simulink model "nonlinearrobot"  (R2020a)
settings: Solver=FixedStepDiscrete  StartTime=0.0  StopTime=1.5  FixedStep=1e-3  RelTol=1e-6  EnableMultiTasking=on
libraries: simulink x1
settings Model: Creator=amal029_old  LastModifiedBy=amal029_old
settings SolverCC: ZeroCrossAlgorithm=Adaptive  AutoInsertRateTranBlk=on  InsertRTBMode=Always
settings DataIOCC: LimitDataPoints=on  ReturnWorkspaceOutputs=off
settings OptimizationCC: LifeSpan=inf
settings DebuggingCC: AllowSymbolicDim=off  SFUnexpectedBacktrackingDiag=warning  SFNoUnconditionalDefaultTransitionDiag=warning  SFExecutionAtInitializationDiag=none  ArithmeticOperatorsInVariantConditions=warning
settings SFSimCC: SimUseLocalCustomCode=off  CustomCodeUndefinedFunction=UseInterfaceOnly
settings RTWCC: RTWUseLocalCustomCode=off
settings CodeAppCC: StateflowObjectComments=on
settings GRTTargetCC: TargetLangStandard=C89/C90 (ANSI)
settings ConfigComp: CovMetricSettings=dw  CovHtmlReporting=on  CovSaveCumulativeToWorkspaceVar=on  CovSaveSingleToWorkspaceVar=on  CovExternalEMLEnable=off  CovSFcnEnable=off

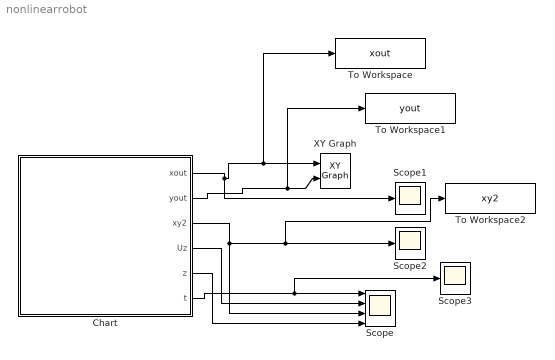
== system nonlinearrobot ==
  Chart : Stateflow chart  TreatAsAtomicUnit=on
  Scope : Scope  NumInputPorts=4
  Scope1 : Scope
  Scope2 : Scope
  Scope3 : Scope
  To Workspace : ToWorkspace  VariableName=xout  SampleTime=-1
  To Workspace1 : ToWorkspace  VariableName=yout  SampleTime=-1
  To Workspace2 : ToWorkspace  VariableName=xy2  SaveFormat=Structure With Time  SampleTime=-1
  XY Graph : simulink/Sinks/XY Graph  xmin=-5  xmax=5  ymin=-5  ymax=5  st=-1
  wires:
  Chart/1(xout) -> Scope1/1, To Workspace/1, XY Graph/1
  Chart/2(yout) -> To Workspace1/1, XY Graph/2
  Chart/3(xy2) -> To Workspace2/1, Scope2/1, Scope/3
  Chart/4(Uz) -> Scope/2
  Chart/5(z) -> Scope/4
  Chart/6(t) -> Scope3/1, Scope/1

== stateflow chart nonlinearrobot/Chart ==
  settings: sampleTime=1e-3
  state Changetheta
    du:
    t = t + v*D;
    z = z + (t)*D;
    en: -log(rand);
  note: This has different Wiener processes, because normrnd is being done separately.
      | These wiener processes are independent.
  state Inner
    du:
    x = x +v*cos(t)*D + v*normrnd(0, sqrt(D));
    y = y + v*sin(t)*D + v*normrnd(0, sqrt(D));
    z = z + x*D*not(x^2+y^2>=v^2);
    xout=x;
    yout=y;
    xy2 = x^2+y^2;
    en: Uz = -log(rand);
  state Move
    du:
    %x = x + v*cos(t)*D + 0.01*normrnd(0, sqrt(D));
    %y = y + v*D*sin(t) + 1*normrnd(0, sqrt(D));
    x = x - v*sin(t)*D*wv + 0*normrnd(0, sqrt(D));
    y = y + v*D*cos(t)*wv + 0*normrnd(0, sqrt(D));
    t = t + wv*D + 0*normrnd(0, sqrt(D));
    xout = x;
    yout = y;
    xy2 = x*x + y*y;
  state Outter
    du:
    x = x + v*cos(t)*D + v*normrnd(0, sqrt(D));
    y = y + v*sin(t)*D + v*normrnd(0, sqrt(D));
    z = z + x*D*not(x^2+y^2 <= v^2);
    xout=x; yout=y;
    xy2=x^2+y^2; z = z + x*D*not(x^2+y^2<=v^2);
    en: Uz = -log(rand);
  Inner -> Changetheta [order 2] : [z >= Uz && not(x^2+y^2>=v^2)]
      | {z=0;t=t;
      | xout=x; yout=y;
      | xy2= x^2+y^2;}
  Changetheta -> Inner [order 1] : [z >= Uz && x^2+y^2<=v^2-e]
      | {z=0;t=t;
      | xout=x;
      | yout=y;
      | xy2 = x^2+y^2;}
  Changetheta -> Outter [order 2] : [z > Uz && x^2+y^2 >= v^2+e]
      | {z=0;
      | t=t;
      | xout=x;
      | yout=y;
      | xy2=x^2+y^2;}
  Outter -> Changetheta [order 2] : [z>=Uz && not(x^2+y^2<=v^2)]
      | {z=0;
      | t=t;
      | xout=x;
      | yout=y;
      | xy2=x^2+y^2;}
  (default) -> Inner [order 1] : [s==2]{x=2; y=1; t=atan(y/x);
      | xout=x; yout=y;
      | xy2=x^2+y^2;z=0;}
  Inner -> Move [order 1] : [x^2+y^2 >= v^2]
      | {t=atan(y/x);xout=x;
      | yout=y;xy2=x^2+y^2;
      | z=0;}
  Move -> Inner [order 1] : [x^2+y^2<=v^2-e]{xout=x;yout=y;xy2=x^2+y^2;
      | t=0;z=0;}
  (default) -> Move [order 3] : {x = 16; xout = x; y = 0; yout = y; t = 0;
      | xy2 = x*x+y*y;z=0;}
  Move -> Outter [order 2] : [x^2+y^2 >= v^2+e]
      | {xout=x; yout=y;
      | xy2=x^2+y^2;t=pi;z=0;}
  Outter -> Move [order 1] : [x^2+y^2<=v^2]
      | {t=atan(y/x);
      | xout=x; yout=y;
      | xy2=x^2+y^2;z=0;}
  (default) -> Outter [order 2] : [s==3]{x=5, y=0;
      | xy2=x^2+y^2;
      | xout=x; yout=y;
      | t=pi;z=0;}
  data: e constant double =1e-1; xout output; yout output; y local; D constant double =1e-3; x local; xy2 output; v constant double =4; wv constant double =0.1; s constant uint8 =2; Uz output; z output; t output
